simulink model "Simulation"  (R2022a)
settings: Solver=FixedStepAuto  StartTime=0.0  StopTime=10  RelTol=1e-3
settings Model: Creator=toker  LastModifiedBy=batua
settings SolverCC: AlgebraicLoopSolver=TrustRegion
settings DataIOCC: ReturnWorkspaceOutputs=off
settings DebuggingCC: UnconnectedInputMsg=warning  UnconnectedOutputMsg=warning  UnconnectedLineMsg=warning  SFMachineParentedDataDiag=warning  ArithmeticOperatorsInVariantConditions=warning
settings SFSimCC: CustomCodeUndefinedFunction=UseInterfaceOnly
settings RTWCC: DLArmComputeVersion=19.05

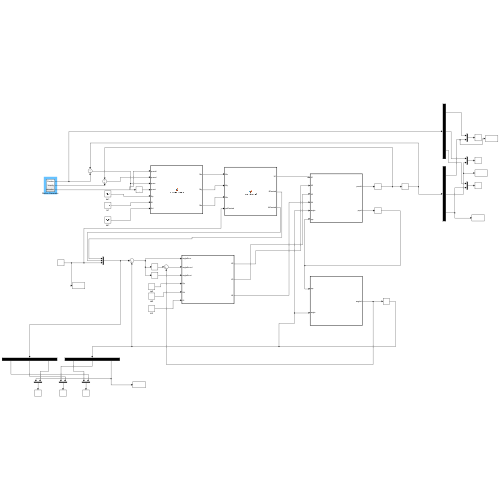
[thumbnail: Simulink's stored preview of the top-level diagram]
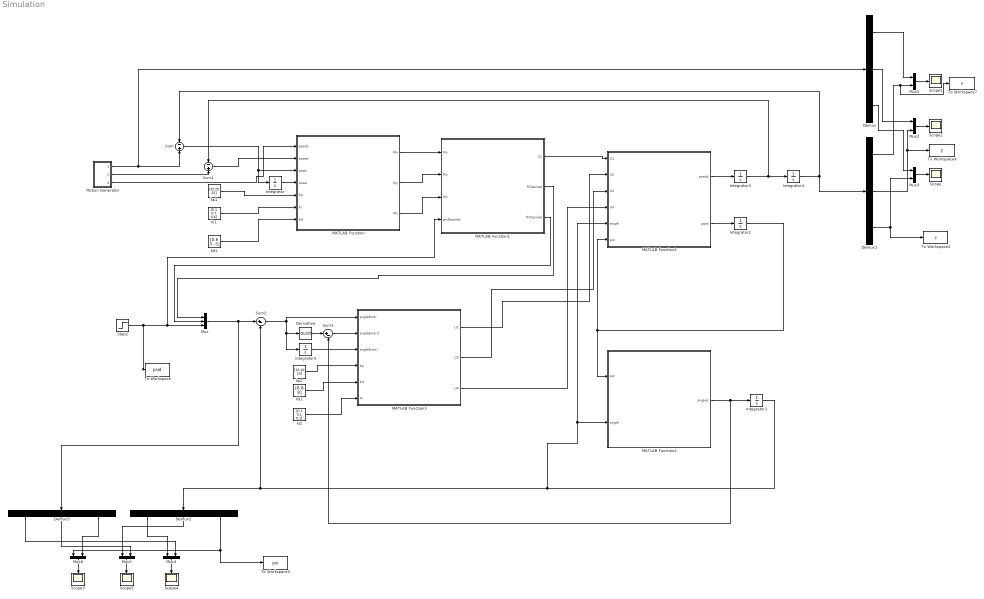
== system Simulation ==
  Demux{,1..3} (4 alike) : Demux  Outputs=3
  Derivative : Derivative
  Integrator{,1..5} (6 alike) : Integrator
  MATLAB Function : MATLAB Function  TreatAsAtomicUnit=on
  MATLAB Function1 : MATLAB Function  TreatAsAtomicUnit=on
  MATLAB Function2 : MATLAB Function  TreatAsAtomicUnit=on
  MATLAB Function3 : MATLAB Function  TreatAsAtomicUnit=on
  MATLAB Function4 : MATLAB Function  TreatAsAtomicUnit=on
  Motion Generator : Subsystem
  Mux : Mux  Inputs=3
  Mux{1..6} (6 alike) : Mux  Inputs=2
  Scope{,1..5} (6 alike) : Scope
  Step2 : Step  After=pi/6  SampleTime=0
  Sum : Sum  Inputs=-|+
  Sum1 : Sum  Inputs=-|+
  Sum2 : Sum  Inputs=|+-
  Sum3 : Sum  Inputs=|+-
  To Workspace : ToWorkspace  VariableName=psid  SaveFormat=Timeseries  SampleTime=-1
  To Workspace2 : ToWorkspace  VariableName=z  SaveFormat=Timeseries  SampleTime=-1
  To Workspace3 : ToWorkspace  VariableName=psi  SaveFormat=Timeseries  SampleTime=-1
  To Workspace4 : ToWorkspace  VariableName=y  SaveFormat=Timeseries  SampleTime=-1
  To Workspace7 : ToWorkspace  VariableName=x  SaveFormat=Timeseries  SampleTime=-1
  kd1 : Constant  Value=[0.6 .5 .5]
  kd2 : Constant  Value=[8 8 8]
  ki1 : Constant  Value=[0.1 0.7 0.6]
  ki2 : Constant  Value=[0.1 0.1 0.1]
  kp1 : Constant  Value=[25 25 25]
  kp2 : Constant  Value=[10 10 10]
  wires:
  Motion Generator/1(Position) -> Demux/1, Sum/2
  Motion Generator/2(Velocity) -> Sum1/2
  kp1/1 -> MATLAB Function/5(Kp)
  kd1/1 -> MATLAB Function/7(Kd)
  ki1/1 -> MATLAB Function/6(Ki)
  Sum/1 -> Integrator/1, MATLAB Function/3(pose)
  Sum1/1 -> MATLAB Function/2(posed)
  Integrator/1 -> MATLAB Function/4(posei)
  MATLAB Function/1(Mx) -> MATLAB Function1/1(Mx)
  MATLAB Function/2(My) -> MATLAB Function1/2(My)
  MATLAB Function/3(Mz) -> MATLAB Function1/3(Mz)
  MATLAB Function4/1(angled) -> Integrator1/1, Sum3/2
  Integrator1/1 -> Demux2/1, Sum2/2, MATLAB Function2/5(angle), MATLAB Function4/2(angle)
  Integrator3/1 -> Integrator4/1, Sum1/1
  MATLAB Function1/2(fiDesired) -> Mux/1
  MATLAB Function1/3(thDesired) -> Mux/2
  Step2/1 -> To Workspace/1, Mux/3, MATLAB Function1/4(psiDesired)
  Mux/1 -> Demux3/1, Sum2/1
  Derivative/1 -> Sum3/1
  Sum3/1 -> MATLAB Function3/2(angleErrord)
  kd2/1 -> MATLAB Function3/5(Kd)
  kp2/1 -> MATLAB Function3/4(Kp)
  Integrator4/1 -> Demux1/1, Sum/1
  MATLAB Function1/1(U1) -> MATLAB Function2/1(U1)
  MATLAB Function3/1(U2) -> MATLAB Function2/2(U2)
  MATLAB Function3/2(U3) -> MATLAB Function2/3(U3)
  MATLAB Function3/3(U4) -> MATLAB Function2/4(U4)
  MATLAB Function2/2(pqrd) -> Integrator2/1
  Sum2/1 -> MATLAB Function3/1(angleError), Integrator5/1, Derivative/1
  ki2/1 -> MATLAB Function3/6(Ki)
  Demux1/1 -> To Workspace7/1, Mux1/2
  Demux/2 -> Mux2/1
  Demux/3 -> Mux3/1
  Demux1/3 -> To Workspace2/1, Mux3/2
  Mux1/1 -> Scope1/1
  Mux2/1 -> Scope2/1
  Mux3/1 -> Scope/1
  Motion Generator/3(Acceleration) -> MATLAB Function/1(posdd)
  MATLAB Function2/1(posdd) -> Integrator3/1
  Mux5/1 -> Scope5/1
  Mux4/1 -> Scope4/1
  Demux2/1 -> Mux4/1
  Demux3/3 -> Mux6/2
  Demux3/2 -> Mux5/2
  Demux2/2 -> Mux5/1
  Demux2/3 -> To Workspace3/1, Mux6/1
  Mux6/1 -> Scope3/1
  Demux3/1 -> Mux4/2
  Integrator5/1 -> MATLAB Function3/3(angleErrori)
  Integrator2/1 -> MATLAB Function2/6(pqr), MATLAB Function4/1(pqr)
  Demux1/2 -> To Workspace4/1, Mux2/2
  Demux/1 -> Mux1/1

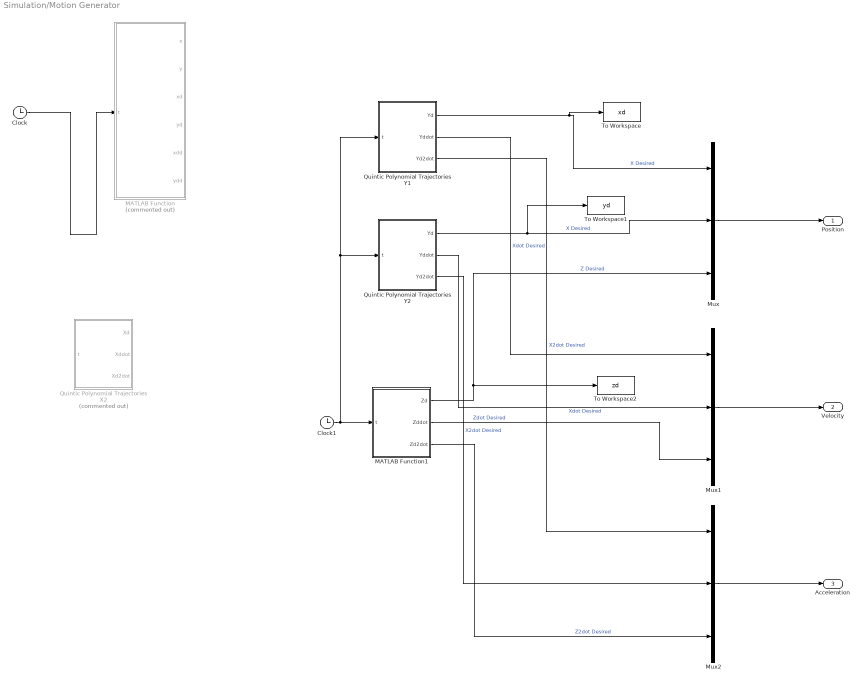
== system Simulation/Motion Generator ==
  Clock : Clock
  Clock1 : Clock
  MATLAB Function : MATLAB Function  Commented=on  TreatAsAtomicUnit=on
  MATLAB Function1 : MATLAB Function  TreatAsAtomicUnit=on
  Mux : Mux  Inputs=3
  Mux1 : Mux  Inputs=3
  Mux2 : Mux  Inputs=3
  Quintic Polynomial Trajectories X2 : MATLAB Function  Commented=on  TreatAsAtomicUnit=on
  Quintic Polynomial Trajectories Y1 : MATLAB Function  TreatAsAtomicUnit=on
  Quintic Polynomial Trajectories Y2 : MATLAB Function  TreatAsAtomicUnit=on
  To Workspace : ToWorkspace  VariableName=xd  SaveFormat=Timeseries  SampleTime=-1
  To Workspace1 : ToWorkspace  VariableName=yd  SaveFormat=Timeseries  SampleTime=-1
  To Workspace2 : ToWorkspace  VariableName=zd  SaveFormat=Timeseries  SampleTime=-1
  Position : Outport  VectorParamsAs1DForOutWhenUnconnected=off
  Velocity : Outport  Port=2  VectorParamsAs1DForOutWhenUnconnected=off
  Acceleration : Outport  Port=3  VectorParamsAs1DForOutWhenUnconnected=off
  wires:
  Mux/1 -> Position/1
  Mux1/1 -> Velocity/1
  Clock/1 -> MATLAB Function/1(t)
  Mux2/1 -> Acceleration/1
  Clock1/1 -> Quintic Polynomial Trajectories Y2/1(t), Quintic Polynomial Trajectories Y1/1(t), MATLAB Function1/1(t)
  MATLAB Function1/1(Zd) -> Mux/3, To Workspace2/1  "Z Desired"
  MATLAB Function1/2(Zddot) -> Mux1/3  "Zdot Desired"
  MATLAB Function1/3(Zd2dot) -> Mux2/3  "Z2dot Desired"
  Quintic Polynomial Trajectories Y1/3(Yd2dot) -> Mux2/1  "X2dot Desired"
  Quintic Polynomial Trajectories Y2/3(Yd2dot) -> Mux2/2  "X2dot Desired"
  Quintic Polynomial Trajectories Y1/1(Yd) -> To Workspace/1, Mux/1  "X Desired"
  Quintic Polynomial Trajectories Y2/1(Yd) -> To Workspace1/1, Mux/2  "X Desired"
  Quintic Polynomial Trajectories Y1/2(Yddot) -> Mux1/1  "Xdot Desired"
  Quintic Polynomial Trajectories Y2/2(Yddot) -> Mux1/2  "Xdot Desired"

== matlab function Simulation/Motion Generator/Quintic Polynomial Trajectories Y2 ==
  data: t input; Yd output; Yddot output; Yd2dot output
function [Yd, Yddot, Yd2dot] = Y_function(t)

t0 = 5;
tf = 10;
 
y0 = 0; 
yf = 10;

vy0 = 0;
vyf = 0;

ay0 = 0;
ayf = 0;

%Ax=b

a = [1 t0 t0^2 t0^3 t0^4 t0^5];
b = [0 1  2*t0 3*t0^2 4*t0^3 5*t0^4];
c = [0 0  2 6*t0 12*t0^2 20*t0^3];
d = [1 tf tf^2 tf^3 tf^4 tf^5];
e = [0 1 2*tf 3*tf^2 4*tf^3 5*tf^4];
f = [0 0 2 6*tf 12*tf^2 20*tf^3];

A_matrix = [ a; b; c; d; e; f ]

b_vector = [ y0; vy0; ay0; yf; vyf; ayf ]

x_vector = inv(A_matrix) * b_vector

if t>=t0 && t<=tf 
 Yd = x_vector(1) + x_vector(2).*t + x_vector(3).*t.^2 + x_vector(4).*t.^3 + x_vector(5).*t.^4 + x_vector(6).*t.^5;
 Yddot = x_vector(2) + 2*x_vector(3).*t + 3*x_vector(4).*t.^2 + 4*x_vector(5).*t.^3 + 5*x_vector(6).*t.^4;
 Yd2dot = 2*x_vector(3) + 6*x_vector(4).*t + 12*x_vector(5).*t.^2 + 20*x_vector(6).*t.^3;
 elseif t>tf
     Yd=yf;
     Yddot=vyf;
     Yd2dot=ayf;
 else
     Yd=0;
     Yddot=0;
     Yd2dot=0;
 end

end

== matlab function Simulation/Motion Generator/Quintic Polynomial Trajectories Y1 ==
  data: t input; Yd output; Yddot output; Yd2dot output
function [Yd, Yddot, Yd2dot] = Y_function(t)

t0 = 5;
tf = 10;
 
y0 = 0; 
yf = 10;

vy0 = 0;
vyf = 0;

ay0 = 0;
ayf = 0;

%Ax=b

a = [1 t0 t0^2 t0^3 t0^4 t0^5];
b = [0 1  2*t0 3*t0^2 4*t0^3 5*t0^4];
c = [0 0  2 6*t0 12*t0^2 20*t0^3];
d = [1 tf tf^2 tf^3 tf^4 tf^5];
e = [0 1 2*tf 3*tf^2 4*tf^3 5*tf^4];
f = [0 0 2 6*tf 12*tf^2 20*tf^3];

A_matrix = [ a; b; c; d; e; f ]

b_vector = [ y0; vy0; ay0; yf; vyf; ayf ]

x_vector = inv(A_matrix) * b_vector

if t>=t0 && t<=tf 
 Yd = x_vector(1) + x_vector(2).*t + x_vector(3).*t.^2 + x_vector(4).*t.^3 + x_vector(5).*t.^4 + x_vector(6).*t.^5;
 Yddot = x_vector(2) + 2*x_vector(3).*t + 3*x_vector(4).*t.^2 + 4*x_vector(5).*t.^3 + 5*x_vector(6).*t.^4;
 Yd2dot = 2*x_vector(3) + 6*x_vector(4).*t + 12*x_vector(5).*t.^2 + 20*x_vector(6).*t.^3;
 elseif t>tf
     Yd=yf;
     Yddot=vyf;
     Yd2dot=ayf;
 else
     Yd=0;
     Yddot=0;
     Yd2dot=0;
 end

end

== matlab function Simulation/Motion Generator/Quintic Polynomial Trajectories X2 ==
  data: t input; Xd output; Xddot output; Xd2dot output
function [Xd, Xddot, Xd2dot]  = X_function(t)

t0 = 0;
tf = 10;
 
x0 = 0;
xf = 0;

vx0 = 0;
vxf = 0;

ax0 = 0;
axf = 0;

%Ax=b

a = [1 t0 t0^2 t0^3 t0^4 t0^5];
b = [0 1  2*t0 3*t0^2 4*t0^3 5*t0^4];
c = [0 0  2 6*t0 12*t0^2 20*t0^3];
d = [1 tf tf^2 tf^3 tf^4 tf^5];
e = [0 1 2*tf 3*tf^2 4*tf^3 5*tf^4];
f = [0 0 2 6*tf 12*tf^2 20*tf^3];

A_matrix = [ a; b; c; d; e; f ]

b_vector = [ x0; vx0; ax0; xf; vxf; axf ]

x_vector = inv(A_matrix) * b_vector

Xd = x_vector(1) + x_vector(2).*t + x_vector(3).*t.^2 + x_vector(4).*t.^3 + x_vector(5).*t.^4 + x_vector(6).*t.^5;
Xddot = x_vector(2) + 2*x_vector(3).*t + 3*x_vector(4).*t.^2 + 4*x_vector(5).*t.^3 + 5*x_vector(6).*t.^4;
Xd2dot = 2*x_vector(3) + 6*x_vector(4).*t + 12*x_vector(5).*t.^2 + 20*x_vector(6).*t.^3;


    if Xd>xf
        Xd=xf;
        Xddot=vxf;
        Xd2dot=axf;
    end
        
end

== matlab function Simulation/Motion Generator/MATLAB Function ==
  data: t input; x output; y output; xd output; yd output; xdd output; ydd output
function [x,y,xd,yd,xdd,ydd] = Source(t)
x = t;
y = 0;


xd = 1;
yd = 0;

xdd= 0;
ydd=0;

== matlab function Simulation/MATLAB Function ==
  data: posdd input size=3; Mx output; posed input; pose input; posei input; Kp input; Ki input; Kd input; My output; Mz output
function [Mx,My,Mz] = positionControl(posdd,posed,pose,posei,Kp,Ki,Kd)
Mx=posdd(1)+Kp(1)*pose(1)+Kd(1)*posed(1)+Ki(1)*posei(1)
My=posdd(2)+Kp(2)*pose(2)+Kd(2)*posed(2)+Ki(2)*posei(2)
Mz=posdd(3)+Kp(3)*pose(3)+Kd(3)*posed(3)+Ki(3)*posei(3)
end

== matlab function Simulation/MATLAB Function1 ==
  data: Mx input; U1 output; My input; Mz input; psiDesired input; fiDesired output; thDesired output
function [U1,fiDesired,thDesired] = virtualControl(Mx,My,Mz,psiDesired)
Ix = 7.5*10^(-3);  % Quadrotor moment of inertia around X axis
Iy = 7.5*10^(-3);  % Quadrotor moment of inertia around Y axis
Iz = 1.3*10^(-2);  % Quadrotor moment of inertia around Z axis
Jr = 6.5*10^(-5);  % Total rotational moment of inertia around the propeller axis
b = 3.13*10^(-5);  % Thrust factor
d = 7.5*10^(-7);  % Drag factor
l = 0.23;  % Distance to the center of the Quadrotor
m = 0.65;  % Mass of the Quadrotor in Kg
g = 9.81;   % Gravitational acceleration
U1= m*sqrt(Mx^2+My^2+(Mz+g)^2);
fiDesired=asin((sin(psiDesired)*Mx-cos(psiDesired)*My)/sqrt(Mx^2+My^2+(Mz+g)^2));
thDesired=asin((cos(psiDesired)*Mx+sin(psiDesired)*My)/(cos(fiDesired)*sqrt(Mx^2+My^2+(Mz+g)^2)));
end

== matlab function Simulation/MATLAB Function2 ==
  data: U1 input; posdd output size=3; U2 input; U3 input; U4 input; angle input; pqrd output size=3; pqr input
function [posdd,pqrd] = quadrotorDynamics(U1,U2,U3,U4,angle,pqr)
% Quadrotor constants
Ix = 7.5*10^(-3);  % Quadrotor moment of inertia around X axis
Iy = 7.5*10^(-3);  % Quadrotor moment of inertia around Y axis
Iz = 1.3*10^(-2);  % Quadrotor moment of inertia around Z axis
Jr = 6.5*10^(-5);  % Total rotational moment of inertia around the propeller axis
b = 3.13*10^(-5);  % Thrust factor
d = 7.5*10^(-7);  % Drag factor
l = 0.23;  % Distance to the center of the Quadrotor
m = 0.65;  % Mass of the Quadrotor in Kg
g = 9.81;   % Gravitational acceleration
fi=angle(1);
th=angle(2);
psi=angle(3);
p=pqr(1);
q=pqr(2);
r=pqr(3);
xdd=(sin(psi)*sin(fi)+cos(psi)*sin(th)*cos(fi))*U1/m;
ydd=(-cos(psi)*sin(fi)+sin(psi)*sin(th)*cos(fi))*U1/m;
zdd=-g+(cos(th)*cos(fi))*U1/m;
pd=(Iy-Iz)/Ix*q*r+U2/Ix;
qd=(Iz-Ix)/Iy*p*r+U3/Iy;
rd=(Ix-Iy)/Iz*p*q+U4/Iz;
posdd=[xdd;ydd;zdd];
pqrd=[pd;qd;rd]
end

== matlab function Simulation/MATLAB Function3 ==
  data: angleError input; U2 output; angleErrord input; angleErrori input; Kp input; Kd input; U3 output; U4 output; Ki input
function [U2,U3,U4] = altitudeControl(angleError,angleErrord,angleErrori,Kp,Kd,Ki)

Ix = 7.5*10^(-3);  % Quadrotor moment of inertia around X axis
Iy = 7.5*10^(-3);  % Quadrotor moment of inertia around Y axis
Iz = 1.3*10^(-2);  % Quadrotor moment of inertia around Z axis
Jr = 6.5*10^(-5);  % Total rotational moment of inertia around the propeller axis
b = 3.13*10^(-5);  % Thrust factor
d = 7.5*10^(-7);  % Drag factor
l = 0.23;  % Distance to the center of the Quadrotor
m = 0.65;  % Mass of the Quadrotor in Kg
g = 9.81;   % Gravitational acceleration
I=[Ix;Iy;Iz];
U2=I(1)*(Kp(1)*angleError(1)+Kd(1)*angleErrord(1)+Ki(1)*angleErrori(1))
U3=I(2)*(Kp(2)*angleError(2)+Kd(2)*angleErrord(2)+Ki(2)*angleErrori(2))
U4=I(3)*(Kp(3)*angleError(3)+Kd(3)*angleErrord(3)+Ki(3)*angleErrori(3))
end

== matlab function Simulation/MATLAB Function4 ==
  data: angled output size=3; pqr input size=3; angle input size=3
function angled  = eulerRate(pqr,angle)

fi=angle(1);
th=angle(2);
psi=angle(3);


angled=[1 sin(fi)*tan(th) cos(fi)*tan(th);
        0 cos(fi)          -sin(fi);
        0 sin(fi)/cos(th) cos(fi)/cos(th)]*pqr;
end

== matlab function Simulation/Motion Generator/MATLAB Function1 ==
  data: t input; Zd output; Zddot output; Zd2dot output
function [Zd, Zddot, Zd2dot] = Z_function(t)


t_i = 0;
t_f = 5;
t_f1 =15; 
 
z_0 = 0;
z_f = 20;
z_f1 = 50;

vz_0 = 0;
vz_f = 0;
vz_f1 = 0;

az_0 = 0;
az_f = 0;
az_f1 = 0;

%Ax=b

if t>t_f && t<=t_f1
    t_i=t_f;  z_0=z_f;  vz_0=vz_f;  az_0=az_f;
    t_f=t_f1; z_f=z_f1; vz_f=vz_f1; az_f=az_f1;
end
    
a = [1 t_i t_i^2 t_i^3 t_i^4 t_i^5];
b = [0 1  2*t_i 3*t_i^2 4*t_i^3 5*t_i^4];
c = [0 0  2 6*t_i 12*t_i^2 20*t_i^3];
d = [1 t_f t_f^2 t_f^3 t_f^4 t_f^5];
e = [0 1 2*t_f 3*t_f^2 4*t_f^3 5*t_f^4];
f = [0 0 2 6*t_f 12*t_f^2 20*t_f^3];


A_matrix = [ a; b; c; d; e; f ];

b_vector = [ z_0; vz_0; az_0; z_f; vz_f; az_f ];

x_vector = inv(A_matrix) * b_vector;

Zd = x_vector(1) + x_vector(2).*t + x_vector(3).*t.^2 + x_vector(4).*t.^3 + x_vector(5).*t.^4 + x_vector(6).*t.^5;
Zddot = x_vector(2) + 2*x_vector(3).*t + 3*x_vector(4).*t.^2 + 4*x_vector(5).*t.^3 + 5*x_vector(6).*t.^4;
Zd2dot = 2*x_vector(3) + 6*x_vector(4).*t + 12*x_vector(5).*t.^2 + 20*x_vector(6).*t.^3;
    if  t>t_f1
        Zd=z_f1;
        Zddot=vz_f1;
        Zd2dot=az_f1;
    end        
end
